simulink subsystem "motores"  (R2023b)
settings: Solver=VariableStepAuto  StartTime=0.0  StopTime=10.0  RelTol=1e-3
libraries: arduinolib x6, simulink x2
settings Model: Creator=Usuario  LastModifiedBy=Usuario

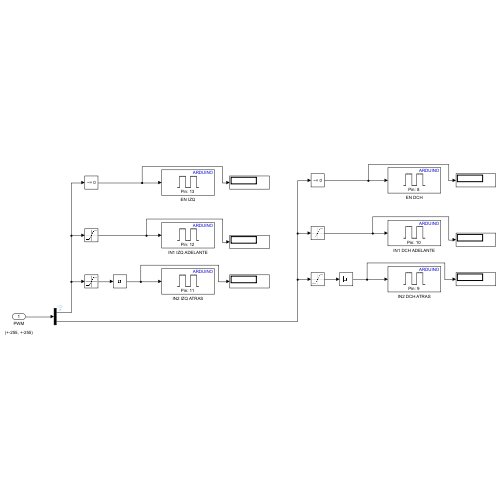
[thumbnail: Simulink's stored preview of the top-level diagram]
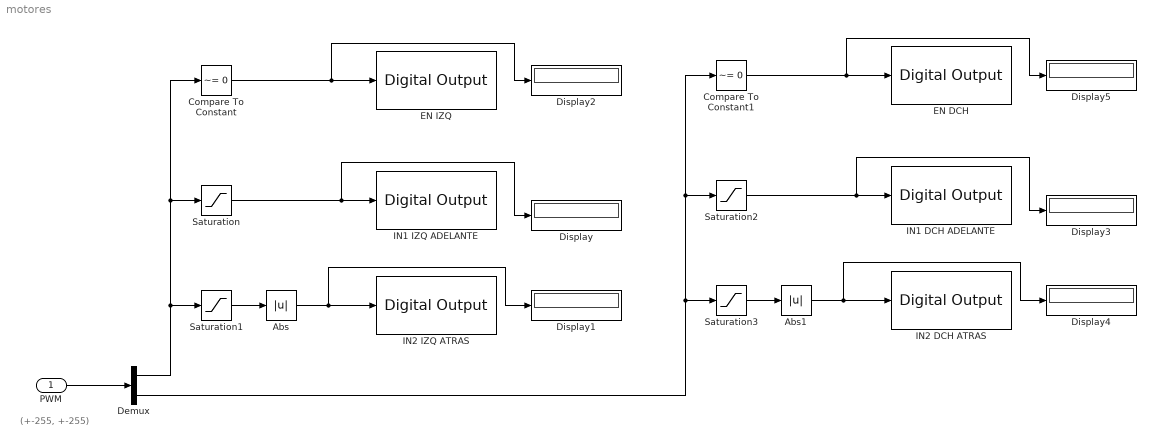
== system motores ==
  note: (+-255, +-255)
  PWM : Inport
  Abs : Abs  SaturateOnIntegerOverflow=off
  Abs1 : Abs  SaturateOnIntegerOverflow=off
  Compare To Constant : simulink/Logic and Bit Operations/Compare To Constant  relop=~=  const=0  OutDataTypeStr=boolean
  Compare To Constant1 : simulink/Logic and Bit Operations/Compare To Constant  relop=~=  const=0  OutDataTypeStr=boolean
  Demux : Demux  Outputs=2
  Display{,1..5} (6 alike) : Display
  EN DCH : arduinolib/Digital Output  pinNumber=8  Direction=output  blockPlatform=arduino
  EN IZQ : arduinolib/Digital Output  pinNumber=13  Direction=output  blockPlatform=arduino
  IN1 DCH ADELANTE : arduinolib/Digital Output  pinNumber=10  Direction=output  blockPlatform=arduino
  IN1 IZQ ADELANTE : arduinolib/Digital Output  pinNumber=11  Direction=output  blockPlatform=arduino
  IN2 DCH ATRAS : arduinolib/Digital Output  pinNumber=9  Direction=output  blockPlatform=arduino
  IN2 IZQ ATRAS : arduinolib/Digital Output  pinNumber=12  Direction=output  blockPlatform=arduino
  Saturation : Saturate  UpperLimit=255  LowerLimit=0
  Saturation1 : Saturate  UpperLimit=0  LowerLimit=-255
  Saturation2 : Saturate  UpperLimit=255  LowerLimit=0
  Saturation3 : Saturate  UpperLimit=0  LowerLimit=-255
  wires:
  PWM/1 -> Demux/1
  Demux/1 -> Saturation1/1, Saturation/1, Compare To Constant/1
  Abs/1 -> Display1/1, IN2 IZQ ATRAS/1
  Compare To Constant/1 -> Display2/1, EN IZQ/1
  Saturation/1 -> Display/1, IN1 IZQ ADELANTE/1
  Saturation1/1 -> Abs/1
  Saturation2/1 -> Display3/1, IN1 DCH ADELANTE/1
  Saturation3/1 -> Abs1/1
  Abs1/1 -> Display4/1, IN2 DCH ATRAS/1
  Compare To Constant1/1 -> Display5/1, EN DCH/1
  Demux/2 -> Saturation3/1, Saturation2/1, Compare To Constant1/1
